simulink model "untitled"  (R2024b)
settings: Solver=VariableStepAuto  StartTime=0.0  StopTime=25  RelTol=1e-3
settings Model: Creator=Noel  LastModifiedBy=Noel

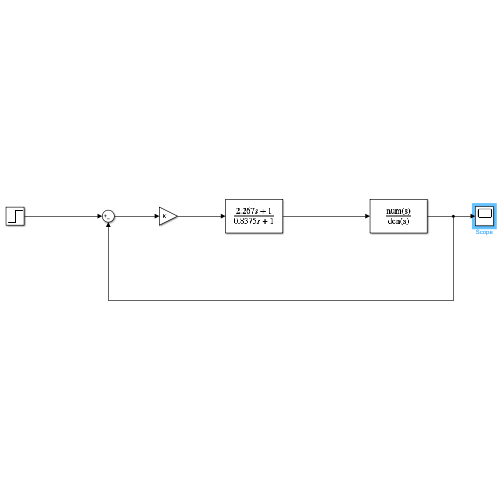
[thumbnail: Simulink's stored preview of the top-level diagram]
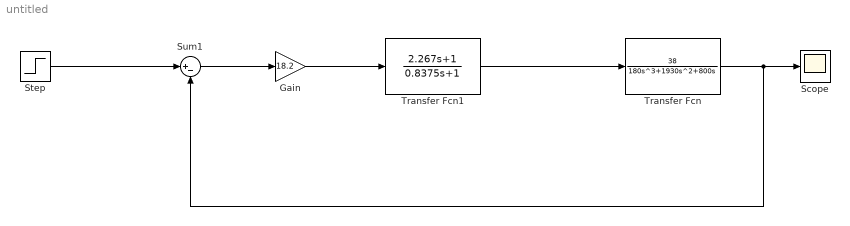
== system untitled ==
  Gain : Gain  Gain=18.2
  Scope : Scope
  Step : Step  SampleTime=0
  Sum1 : Sum  Inputs=|+-
  Transfer Fcn : TransferFcn  Numerator=[38]  Denominator=[180 1930 800 0]
  Transfer Fcn1 : TransferFcn  Numerator=[2.267 1]  Denominator=[0.8375 1]
  wires:
  Transfer Fcn/1 -> Sum1/2, Scope/1
  Step/1 -> Sum1/1
  Transfer Fcn1/1 -> Transfer Fcn/1
  Gain/1 -> Transfer Fcn1/1
  Sum1/1 -> Gain/1
